simulink model "schemaControlloDinamicaInversa"  (Simulink 8.1)
settings: Solver=ode45  StartTime=0.0  StopTime=20  FixedStep=0.001  MaxStep=0.004  RelTol=1e-3
undefined symbols (not defined in the file): DinamicaDiretta, q0
CloseFcn:
  | rtwprivate ssgencode ModelCloseRequest ContributiCoppieComau
settings Model: Creator=Alessandro  LastModifiedBy=alessandro  ExtModeAutoUpdateStatusClock=off
settings SolverCC: AlgebraicLoopSolver=LineSearch
settings OptimizationCC: InitFltsAndDblsToZero=on
settings DebuggingCC: SaveWithParameterizedLinksMsg=none  SignalResolutionControl=TryResolveAllWithWarning  InheritedTsInSrcMsg=none  DiscreteInheritContinuousMsg=none  MultiTaskDSMMsg=warning  MultiTaskCondExecSysMsg=none  TasksWithSamePriorityMsg=none
settings GRTTargetCC: TargetFcnLib=ansi_tfl_tmw.mat  CodeReplacementLibrary=None  CPPClassGenCompliant=on

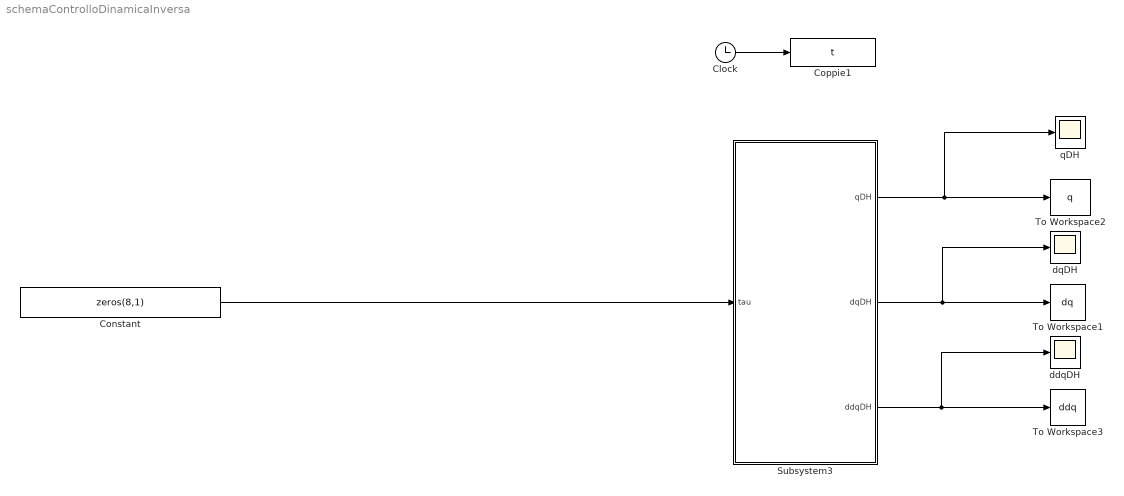
== system schemaControlloDinamicaInversa ==
  Clock : Clock
  Constant : Constant  Value=zeros(8,1)
  Coppie1 : ToWorkspace  VariableName=t  SampleTime=-1
  Subsystem3 : Subsystem
      mask Display:
      | disp('Manipolatore');
      | port_label('input', 1, 'tau');
      | port_label('output', 1, 'qDH');
      | port_label('output', 2, 'dqDH');
      | port_label('output', 3, 'ddqDH');
  To Workspace1 : ToWorkspace  VariableName=dq  SampleTime=-1
  To Workspace2 : ToWorkspace  VariableName=q  SampleTime=-1
  To Workspace3 : ToWorkspace  VariableName=ddq  SampleTime=-1
  ddqDH : Scope
      settings: SaveName=ScopeData2
  dqDH : Scope
  qDH : Scope
  wires:
  Clock/1 -> Coppie1/1
  Subsystem3/2(dqDH) -> dqDH/1, To Workspace1/1
  Subsystem3/1(qDH) -> qDH/1, To Workspace2/1
  Subsystem3/3(ddqDH) -> To Workspace3/1, ddqDH/1
  Constant/1 -> Subsystem3/1(tau)

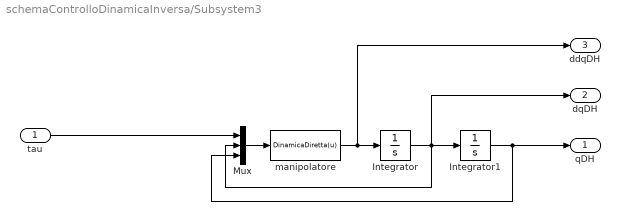
== system schemaControlloDinamicaInversa/Subsystem3 ==
  tau : Inport
  Integrator : Integrator  InitialCondition=zeros(8,1)
  Integrator1 : Integrator  InitialCondition=q0
  Mux : Mux  Inputs=3
  manipolatore : MATLABFcn  MATLABFcn=DinamicaDiretta(u)
  qDH : Outport
  dqDH : Outport  Port=2
  ddqDH : Outport  Port=3
  wires:
  Mux/1 -> manipolatore/1
  manipolatore/1 -> ddqDH/1, Integrator/1
  Integrator/1 -> dqDH/1, Mux/2, Integrator1/1
  Integrator1/1 -> Mux/3, qDH/1
  tau/1 -> Mux/1
